simulink model "simple_adder"  (R2022a)
settings: Solver=VariableStepAuto  StartTime=0.0  StopTime=10.0  RelTol=1e-3
settings Model: Creator=Home computer  LastModifiedBy=Home computer

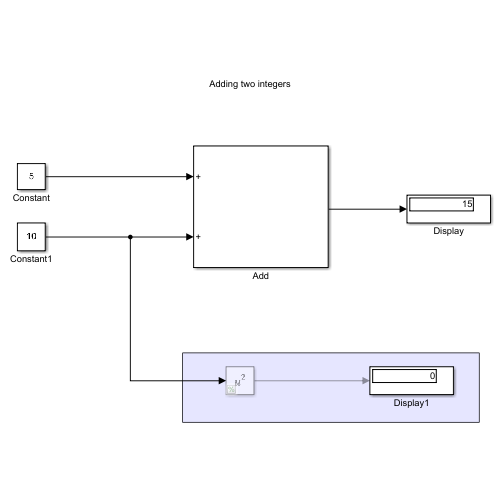
[thumbnail: Simulink's stored preview of the top-level diagram]
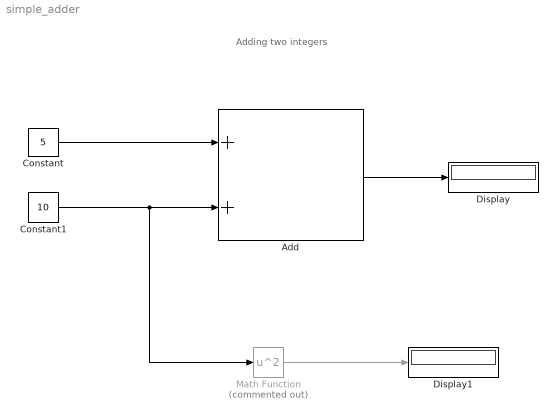
== system simple_adder ==
  note: Adding two integers
  Add : Sum
  Constant : Constant  Value=5
  Constant1 : Constant  Value=10
  Display : Display
  Display1 : Display
  Math Function : Math  Commented=on  Operator=square
  wires:
  Constant/1 -> Add/1
  Constant1/1 -> Math Function/1, Add/2
  Add/1 -> Display/1
  Math Function/1 -> Display1/1
